simulink model "bh_proto_TQ_FFWD"  (R2016b)
settings: Solver=ode23s  StartTime=0.0  StopTime=60  FixedStep=0.001  RelTol=1e-5  EnableMultiTasking=on
undefined symbols (not defined in the file or in its folder): b1_damp, b2_damp, b3_damp, b4_damp, g, L1x, L1y, L1z, L2x, L2y, L2z, L3x, L3y, L3z, mass1, mass2, mass3, mass4, Rturn, TH1, TH1_D, TH1_DD, TH2, TH2_D, TH2_DD, TH3, TH3_D, TH3_DD, TH4, TH4_D, TH4_DD, theta1_0, theta1_dot_0, theta2_0, theta2_dot_0, theta3_0, theta3_dot_0, theta4_0, theta4_dot_0
libraries: simulink_extras x34, simulink x11, discretizing x8
(part 1 of 3)
settings Model: SimulationMode=rapid-accelerator  Creator=bhorton  LastModifiedBy=bhorton
settings SolverCC: ZeroCrossAlgorithm=Adaptive
settings OptimizationCC: LifeSpan=inf
settings DebuggingCC: SFUnexpectedBacktrackingDiag=warning  SFNoUnconditionalDefaultTransitionDiag=warning  SFExecutionAtInitializationDiag=none
settings GRTTargetCC: TargetLangStandard=C89/C90 (ANSI)
settings ConfigComp: CovMetricSettings=dw  CovHtmlReporting=on  CovSaveCumulativeToWorkspaceVar=on  CovSaveSingleToWorkspaceVar=on  CovExternalEMLEnable=off
settings SimscapeCC: SimscapeLogDataHistory=10000  SelectedTab=General

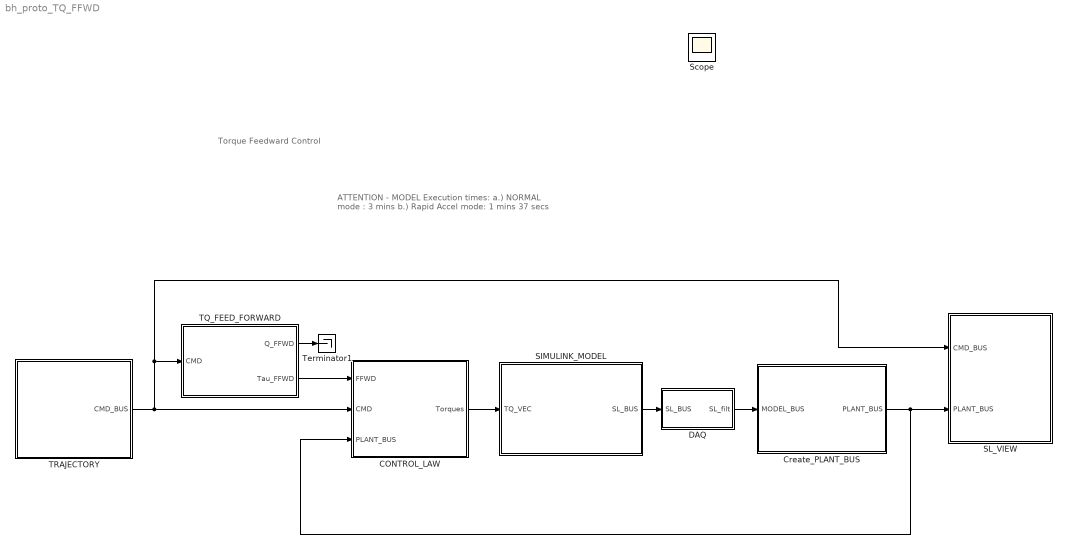
== system bh_proto_TQ_FFWD ==
  note: Torque Feedward Control
  note: ATTENTION - MODEL Execution times:
      | a.) NORMAL mode : 3 mins
      | b.) Rapid Accel mode: 1 mins 37 secs
  CONTROL_LAW : Subsystem
  Create_PLANT_BUS : Subsystem
  DAQ : Subsystem
  SIMULINK_MODEL : Subsystem
  SL_VIEW : Subsystem
  TQ_FEED_FORWARD : Subsystem
  TRAJECTORY : Subsystem
  Terminator1 : Terminator
  Scope : Scope
  wires:
  TRAJECTORY/1(CMD_BUS) -> SL_VIEW/1(CMD_BUS), TQ_FEED_FORWARD/1(CMD), CONTROL_LAW/2(CMD)
  Create_PLANT_BUS/1(PLANT_BUS) -> SL_VIEW/2(PLANT_BUS), CONTROL_LAW/3(PLANT_BUS)
  SIMULINK_MODEL/1(SL_BUS) -> DAQ/1(SL_BUS)
  CONTROL_LAW/1(Torques) -> SIMULINK_MODEL/1(TQ_VEC)
  TQ_FEED_FORWARD/2(Tau_FFWD) -> CONTROL_LAW/1(FFWD)
  TQ_FEED_FORWARD/1(Q_FFWD) -> Terminator1/1
  DAQ/1(SL_filt) -> Create_PLANT_BUS/1(MODEL_BUS)

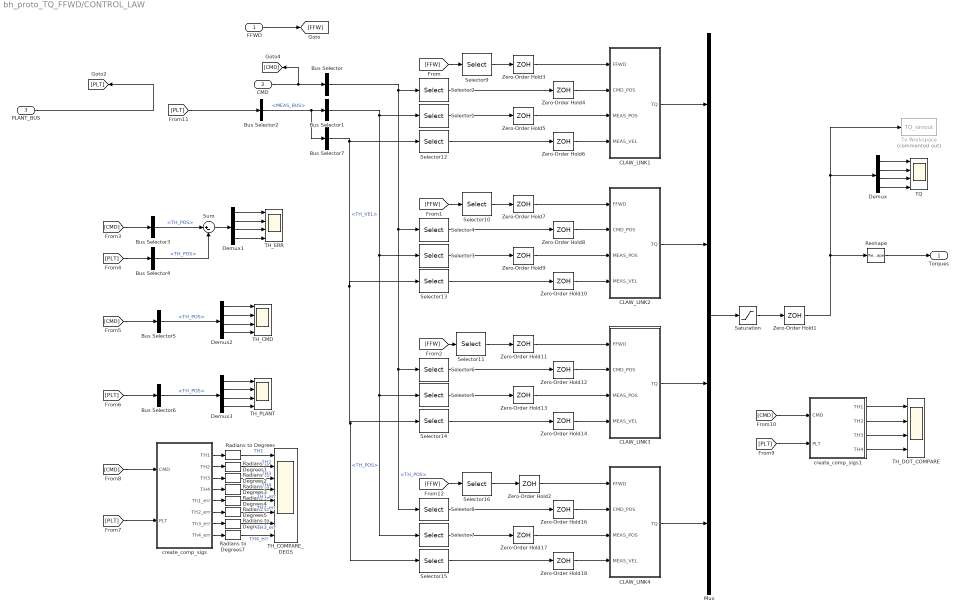
== system bh_proto_TQ_FFWD/CONTROL_LAW ==
  FFWD : Inport
  CMD : Inport  Port=2
  PLANT_BUS : Inport  Port=3
  Bus Selector{,1,3,5} (4 alike) : BusSelector  OutputSignals=TH_POS
  Bus Selector2 : BusSelector  OutputSignals=MEAS_BUS
  Bus Selector4 : BusSelector  OutputSignals=MEAS_BUS.TH_POS
  Bus Selector6 : BusSelector  OutputSignals=MEAS_BUS.TH_POS
  Bus Selector7 : BusSelector  OutputSignals=TH_VEL
  CLAW_LINK1 : Subsystem
  CLAW_LINK2 : Subsystem
  CLAW_LINK3 : Subsystem
  CLAW_LINK4 : Subsystem
  Demux{,1..3} (4 alike) : Demux
  Mux : Mux
  Radians to Degrees{,1..7} (8 alike) : simulink_extras/Transformations/Radians to Degrees
  Reshape : Reshape  OutputDimensionality=Column vector (2-D)
  Saturation : Saturate  UpperLimit=3  LowerLimit=-3
  Selector{1..2,9,12} (4 alike) : Selector  InputPortWidth=4  IndexOptions=Index vector (dialog)  Indices=1  OutputSizes=1
  Selector{3..4,10,13} (4 alike) : Selector  InputPortWidth=4  IndexOptions=Index vector (dialog)  Indices=2  OutputSizes=1
  Selector{5..6,11,14} (4 alike) : Selector  InputPortWidth=4  IndexOptions=Index vector (dialog)  Indices=3  OutputSizes=1
  Selector{7..8,15..16} (4 alike) : Selector  InputPortWidth=4  IndexOptions=Index vector (dialog)  Indices=4  OutputSizes=1
  Sum : Sum  Inputs=|+-
  TH_CMD : Scope  NumInputPorts=4
  TH_COMPARE_DEGS : Scope  NumInputPorts=8
  TH_DOT_COMPARE : Scope  NumInputPorts=4
  TH_ERR : Scope  NumInputPorts=4
  TH_PLANT : Scope  NumInputPorts=4
  TQ : Scope  NumInputPorts=4
  To Workspace : ToWorkspace  Commented=on  VariableName=TQ_simout  SaveFormat=Structure With Time  SampleTime=-1
  Zero-Order Hold{1..14,16..18} (17 alike) : ZeroOrderHold  SampleTime=0.001
      settings: AttributesFormatString=DT =%<SampleTime>
  create_comp_sigs : Subsystem
  create_comp_sigs1 : Subsystem
  Torques : Outport
  wires:
  Mux/1 -> Saturation/1
  Selector9/1 -> Zero-Order Hold3/1
  CMD/1 -> [CMD], Bus Selector/1
  Selector1/1 -> Zero-Order Hold5/1
  Selector2/1 -> Zero-Order Hold4/1
  Bus Selector/1 -> Selector8/1, Selector6/1, Selector4/1, Selector2/1  "<TH_POS>"
  Bus Selector1/1 -> Selector5/1, Selector7/1, Selector3/1, Selector1/1  "<TH_POS>"
  Bus Selector2/1 -> Bus Selector7/1, Bus Selector1/1  "<MEAS_BUS>"
  Demux/1 -> TQ/1
  Demux/2 -> TQ/2
  Demux/4 -> TQ/4
  Demux/3 -> TQ/3
  FFWD/1 -> [FFW]
  [FFW] -> Selector9/1
  [FFW] -> Selector10/1
  [FFW] -> Selector11/1
  Demux1/1 -> TH_ERR/1
  Demux1/2 -> TH_ERR/2
  Demux1/4 -> TH_ERR/4
  Demux1/3 -> TH_ERR/3
  PLANT_BUS/1 -> [PLT]
  [CMD] -> Bus Selector3/1
  [PLT] -> Bus Selector4/1
  Bus Selector3/1 -> Sum/1  "<TH_POS>"
  Bus Selector4/1 -> Sum/2  "<TH_POS>"
  Sum/1 -> Demux1/1
  Demux2/1 -> TH_CMD/1
  Demux2/2 -> TH_CMD/2
  Demux2/4 -> TH_CMD/4
  Demux2/3 -> TH_CMD/3
  [CMD] -> Bus Selector5/1
  Bus Selector5/1 -> Demux2/1  "<TH_POS>"
  Demux3/1 -> TH_PLANT/1
  Demux3/2 -> TH_PLANT/2
  Demux3/4 -> TH_PLANT/4
  Demux3/3 -> TH_PLANT/3
  [PLT] -> Bus Selector6/1
  Bus Selector6/1 -> Demux3/1  "<TH_POS>"
  Bus Selector7/1 -> Selector15/1, Selector14/1, Selector13/1, Selector12/1  "<TH_VEL>"
  Selector12/1 -> Zero-Order Hold6/1
  CLAW_LINK4/1(TQ) -> Mux/4
  CLAW_LINK3/1(TQ) -> Mux/3
  CLAW_LINK2/1(TQ) -> Mux/2
  CLAW_LINK1/1(TQ) -> Mux/1
  Saturation/1 -> Zero-Order Hold1/1
  Zero-Order Hold3/1 -> CLAW_LINK1/1(FFWD)
  Zero-Order Hold4/1 -> CLAW_LINK1/2(CMD_POS)
  Zero-Order Hold5/1 -> CLAW_LINK1/3(MEAS_POS)
  Zero-Order Hold6/1 -> CLAW_LINK1/4(MEAS_VEL)
  Selector10/1 -> Zero-Order Hold7/1
  Selector3/1 -> Zero-Order Hold9/1
  Selector4/1 -> Zero-Order Hold8/1
  Selector13/1 -> Zero-Order Hold10/1
  Zero-Order Hold7/1 -> CLAW_LINK2/1(FFWD)
  Zero-Order Hold8/1 -> CLAW_LINK2/2(CMD_POS)
  Zero-Order Hold9/1 -> CLAW_LINK2/3(MEAS_POS)
  Zero-Order Hold10/1 -> CLAW_LINK2/4(MEAS_VEL)
  Selector5/1 -> Zero-Order Hold13/1
  Selector6/1 -> Zero-Order Hold12/1
  Selector14/1 -> Zero-Order Hold14/1
  Zero-Order Hold11/1 -> CLAW_LINK3/1(FFWD)
  Zero-Order Hold12/1 -> CLAW_LINK3/2(CMD_POS)
  Zero-Order Hold13/1 -> CLAW_LINK3/3(MEAS_POS)
  Zero-Order Hold14/1 -> CLAW_LINK3/4(MEAS_VEL)
  Selector11/1 -> Zero-Order Hold11/1
  Selector7/1 -> Zero-Order Hold17/1
  Selector8/1 -> Zero-Order Hold16/1
  Selector15/1 -> Zero-Order Hold18/1
  Zero-Order Hold16/1 -> CLAW_LINK4/2(CMD_POS)
  Zero-Order Hold17/1 -> CLAW_LINK4/3(MEAS_POS)
  Zero-Order Hold18/1 -> CLAW_LINK4/4(MEAS_VEL)
  Zero-Order Hold2/1 -> CLAW_LINK4/1(FFWD)
  [PLT] -> create_comp_sigs/2(PLT)
  [CMD] -> create_comp_sigs/1(CMD)
  create_comp_sigs/1(TH1) -> Radians to Degrees/1
  create_comp_sigs/2(TH2) -> Radians to Degrees1/1
  create_comp_sigs/3(TH3) -> Radians to Degrees2/1
  create_comp_sigs/4(TH4) -> Radians to Degrees3/1
  [PLT] -> create_comp_sigs1/2(PLT)
  [CMD] -> create_comp_sigs1/1(CMD)
  create_comp_sigs1/1(TH1) -> TH_DOT_COMPARE/1
  create_comp_sigs1/2(TH2) -> TH_DOT_COMPARE/2
  create_comp_sigs1/3(TH3) -> TH_DOT_COMPARE/3
  create_comp_sigs1/4(TH4) -> TH_DOT_COMPARE/4
  Zero-Order Hold1/1 -> Reshape/1, To Workspace/1, Demux/1
  [PLT] -> Bus Selector2/1
  [FFW] -> Selector16/1
  Selector16/1 -> Zero-Order Hold2/1
  create_comp_sigs/5(Th1_err) -> Radians to Degrees4/1
  create_comp_sigs/6(TH2_err) -> Radians to Degrees5/1
  create_comp_sigs/7(Th3_err) -> Radians to Degrees6/1
  create_comp_sigs/8(Th4_err) -> Radians to Degrees7/1
  Radians to Degrees7/1 -> TH_COMPARE_DEGS/8  "TH4_err"
  Radians to Degrees6/1 -> TH_COMPARE_DEGS/7  "TH3_err"
  Radians to Degrees5/1 -> TH_COMPARE_DEGS/6  "TH2_err"
  Radians to Degrees4/1 -> TH_COMPARE_DEGS/5  "TH1_err"
  Radians to Degrees3/1 -> TH_COMPARE_DEGS/4  "TH4"
  Radians to Degrees2/1 -> TH_COMPARE_DEGS/3  "TH3"
  Radians to Degrees1/1 -> TH_COMPARE_DEGS/2  "TH2"
  Radians to Degrees/1 -> TH_COMPARE_DEGS/1  "TH1"
  Reshape/1 -> Torques/1

== system bh_proto_TQ_FFWD/Create_PLANT_BUS ==
  MODEL_BUS : Inport
  CALC_BUS : Subsystem
  MEAS : Subsystem
  Subsystem : Subsystem
  Subsystem1 : Subsystem
  PLANT_BUS : Outport
  wires:
  MODEL_BUS/1 -> MEAS/1(MODEL_BUS), CALC_BUS/1(MODEL_BUS), Subsystem/1(MODEL)
  Subsystem/1(PLANT_B) -> PLANT_BUS/1
  CALC_BUS/1(CALC_POS) -> Subsystem1/1(POS), Subsystem/3(CALC_POS)
  MEAS/1(MEAS) -> Subsystem/2(MEAS)
  Subsystem1/1(GTQ) -> Subsystem/4(CALC_GRAV_TQ)

== system bh_proto_TQ_FFWD/DAQ ==
  SL_BUS : Inport
  Bus Assignment : BusAssignment  AssignedSignals=TH1,TH2,TH3,TH4,TH1_D,TH2_D,TH3_D,TH4_D,TH1_DD,TH2_DD,TH3_DD,TH4_DD
  Bus Selector : BusSelector  OutputSignals=TH1,TH2,TH3,TH4
  Bus Selector1 : BusSelector  OutputSignals=TH1_D,TH2_D,TH3_D,TH4_D
  Bus Selector2 : BusSelector  OutputSignals=TH1_DD,TH2_DD,TH3_DD,TH4_DD
  Demux : Demux
  Demux1 : Demux
  Demux2 : Demux
  LPF : Subsystem  mask{fc=100}
      mask prompts: fc "LPF cutoff Frequency (Hz)"
      mask Display: fprintf('LPF\n fc = %.0f (Hz)', fc);
  Mux : Mux
  Mux1 : Mux
  Mux2 : Mux
  SL_filt : Outport
  wires:
  Bus Selector/1 -> Mux/1  "<TH1>"
  Bus Selector/2 -> Mux/2  "<TH2>"
  Bus Selector/3 -> Mux/3  "<TH3>"
  Bus Selector/4 -> Mux/4  "<TH4>"
  Bus Selector1/1 -> Mux1/1  "<TH1_D>"
  Bus Selector1/2 -> Mux1/2  "<TH2_D>"
  Bus Selector1/3 -> Mux1/3  "<TH3_D>"
  Bus Selector1/4 -> Mux1/4  "<TH4_D>"
  Bus Selector2/1 -> Mux2/1  "<TH1_DD>"
  Bus Selector2/2 -> Mux2/2  "<TH2_DD>"
  Bus Selector2/3 -> Mux2/3  "<TH3_DD>"
  Bus Selector2/4 -> Mux2/4  "<TH4_DD>"
  Mux1/1 -> LPF/2(TH_D)
  Mux/1 -> LPF/1(TH)
  Mux2/1 -> LPF/3(TH_DD)
  LPF/1(TH_filt) -> Demux/1
  LPF/2(TH_D_filt) -> Demux1/1
  LPF/3(TH_DD_filt) -> Demux2/1
  SL_BUS/1 -> [A], Bus Selector2/1, Bus Selector/1, Bus Selector1/1
  [A] -> Bus Assignment/1
  Demux/1 -> Bus Assignment/2
  Demux/2 -> Bus Assignment/3
  Demux/3 -> Bus Assignment/4
  Demux/4 -> Bus Assignment/5
  Demux1/1 -> Bus Assignment/6
  Demux1/2 -> Bus Assignment/7
  Demux1/3 -> Bus Assignment/8
  Demux1/4 -> Bus Assignment/9
  Demux2/1 -> Bus Assignment/10
  Demux2/2 -> Bus Assignment/11
  Demux2/3 -> Bus Assignment/12
  Demux2/4 -> Bus Assignment/13
  Bus Assignment/1 -> SL_filt/1

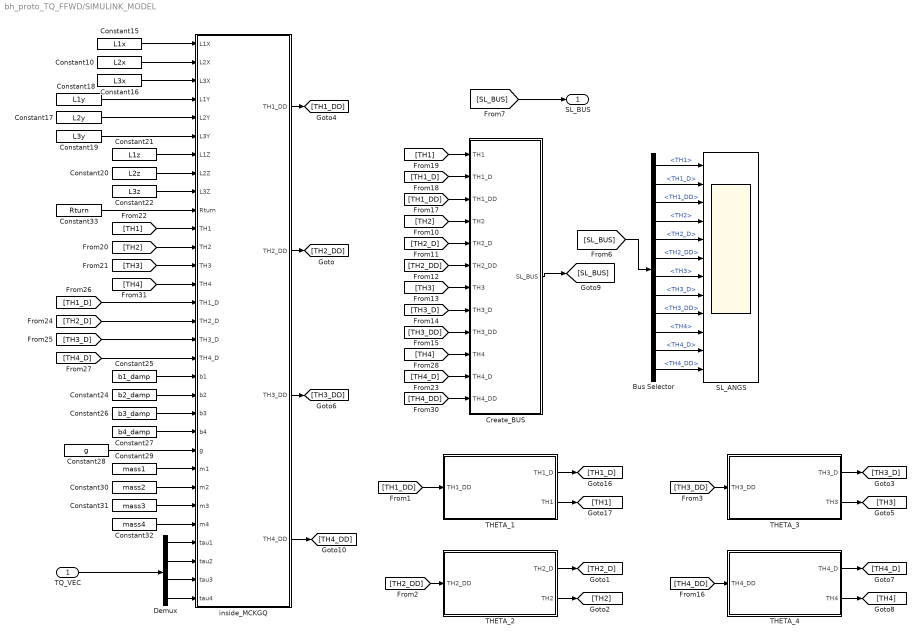
== system bh_proto_TQ_FFWD/SIMULINK_MODEL ==
  TQ_VEC : Inport
  Bus Selector : BusSelector  OutputSignals=TH1,TH1_D,TH1_DD,TH2,TH2_D,TH2_DD,TH3,TH3_D,TH3_DD,TH4,TH4_D,TH4_DD
  Constant10 : Constant  Value=L2x
  Constant15 : Constant  Value=L1x
  Constant16 : Constant  Value=L3x
  Constant17 : Constant  Value=L2y
  Constant18 : Constant  Value=L1y
  Constant19 : Constant  Value=L3y
  Constant20 : Constant  Value=L2z
  Constant21 : Constant  Value=L1z
  Constant22 : Constant  Value=L3z
  Constant24 : Constant  Value=b2_damp
  Constant25 : Constant  Value=b1_damp
  Constant26 : Constant  Value=b3_damp
  Constant27 : Constant  Value=b4_damp
  Constant28 : Constant  Value=g
  Constant29 : Constant  Value=mass1
  Constant30 : Constant  Value=mass2
  Constant31 : Constant  Value=mass3
  Constant32 : Constant  Value=mass4
  Constant33 : Constant  Value=Rturn
  Create_BUS : Subsystem
  Demux : Demux
  SL_ANGS : Scope  NumInputPorts=12
  THETA_1 : Subsystem
  THETA_2 : Subsystem
  THETA_3 : Subsystem
  THETA_4 : Subsystem
  inside_MCKGQ : Subsystem
  SL_BUS : Outport
  wires:
  [SL_BUS] -> Bus Selector/1
  [SL_BUS] -> SL_BUS/1
  Create_BUS/1(SL_BUS) -> [SL_BUS]
  Bus Selector/2 -> SL_ANGS/2  "<TH1_D>"
  Bus Selector/3 -> SL_ANGS/3  "<TH1_DD>"
  Bus Selector/1 -> SL_ANGS/1  "<TH1>"
  Bus Selector/4 -> SL_ANGS/4  "<TH2>"
  Bus Selector/5 -> SL_ANGS/5  "<TH2_D>"
  Bus Selector/6 -> SL_ANGS/6  "<TH2_DD>"
  Bus Selector/7 -> SL_ANGS/7  "<TH3>"
  Bus Selector/8 -> SL_ANGS/8  "<TH3_D>"
  Bus Selector/9 -> SL_ANGS/9  "<TH3_DD>"
  [TH2_DD] -> THETA_2/1(TH2_DD)
  THETA_2/2(TH2) -> [TH2]
  THETA_2/1(TH2_D) -> [TH2_D]
  [TH1_DD] -> THETA_1/1(TH1_DD)
  THETA_1/1(TH1_D) -> [TH1_D]
  THETA_1/2(TH1) -> [TH1]
  inside_MCKGQ/2(TH2_DD) -> [TH2_DD]
  [TH3_DD] -> THETA_3/1(TH3_DD)
  THETA_3/2(TH3) -> [TH3]
  THETA_3/1(TH3_D) -> [TH3_D]
  inside_MCKGQ/1(TH1_DD) -> [TH1_DD]
  inside_MCKGQ/3(TH3_DD) -> [TH3_DD]
  [TH3_DD] -> Create_BUS/9(TH3_DD)
  [TH1] -> Create_BUS/1(TH1)
  [TH1_D] -> Create_BUS/2(TH1_D)
  [TH1_DD] -> Create_BUS/3(TH1_DD)
  [TH2] -> Create_BUS/4(TH2)
  [TH2_D] -> Create_BUS/5(TH2_D)
  [TH2_DD] -> Create_BUS/6(TH2_DD)
  [TH3] -> Create_BUS/7(TH3)
  [TH3_D] -> Create_BUS/8(TH3_D)
  [TH4_DD] -> THETA_4/1(TH4_DD)
  THETA_4/2(TH4) -> [TH4]
  THETA_4/1(TH4_D) -> [TH4_D]
  [TH2] -> inside_MCKGQ/12(TH2)
  [TH3] -> inside_MCKGQ/13(TH3)
  [TH1] -> inside_MCKGQ/11(TH1)
  Constant10/1 -> inside_MCKGQ/2(L2X)
  Constant16/1 -> inside_MCKGQ/3(L3X)
  Constant15/1 -> inside_MCKGQ/1(L1X)
  Constant19/1 -> inside_MCKGQ/6(L3Y)
  Constant17/1 -> inside_MCKGQ/5(L2Y)
  Constant18/1 -> inside_MCKGQ/4(L1Y)
  Constant22/1 -> inside_MCKGQ/9(L3Z)
  Constant20/1 -> inside_MCKGQ/8(L2Z)
  Constant21/1 -> inside_MCKGQ/7(L1Z)
  [TH1_D] -> inside_MCKGQ/15(TH1_D)
  [TH2_D] -> inside_MCKGQ/16(TH2_D)
  [TH3_D] -> inside_MCKGQ/17(TH3_D)
  [TH4_D] -> inside_MCKGQ/18(TH4_D)
  Constant25/1 -> inside_MCKGQ/19(b1)
  Constant24/1 -> inside_MCKGQ/20(b2)
  Constant26/1 -> inside_MCKGQ/21(b3)
  Constant27/1 -> inside_MCKGQ/22(b4)
  Constant28/1 -> inside_MCKGQ/23(g)
  Constant29/1 -> inside_MCKGQ/24(m1)
  Constant30/1 -> inside_MCKGQ/25(m2)
  Constant31/1 -> inside_MCKGQ/26(m3)
  Constant32/1 -> inside_MCKGQ/27(m4)
  Constant33/1 -> inside_MCKGQ/10(Rturn)
  [TH4_D] -> Create_BUS/11(TH4_D)
  [TH4_DD] -> Create_BUS/12(TH4_DD)
  [TH4] -> Create_BUS/10(TH4)
  [TH4] -> inside_MCKGQ/14(TH4)
  inside_MCKGQ/4(TH4_DD) -> [TH4_DD]
  Bus Selector/10 -> SL_ANGS/10  "<TH4>"
  Bus Selector/11 -> SL_ANGS/11  "<TH4_D>"
  Bus Selector/12 -> SL_ANGS/12  "<TH4_DD>"
  Demux/2 -> inside_MCKGQ/29(tau2)
  Demux/3 -> inside_MCKGQ/30(tau3)
  Demux/4 -> inside_MCKGQ/31(tau4)
  TQ_VEC/1 -> Demux/1
  Demux/1 -> inside_MCKGQ/28(tau1)

== system bh_proto_TQ_FFWD/SL_VIEW ==
  CMD_BUS : Inport
  PLANT_BUS : Inport  Port=2
  Bus Selector4 : BusSelector  OutputSignals=CALC_POS_BUS.WF_pos_EFF
  COMPARE_XYZ_EFF (mm) COMPARE_THETA (degs) : Scope  NumInputPorts=16
  Demux : Demux  Outputs=3
  Gain{,1..5} (6 alike) : Gain  Gain=1000
  Ground : Ground
  Ground1 : Ground
  MODEL_MATH_SL : simulink/Sinks/XY Graph  xmin=0  xmax=1.6  ymin=0  ymax=1.6  st=-1
  PLANT_XYZ_EFF : Scope  NumInputPorts=3
  Radians to Degrees{,1..7} (8 alike) : simulink_extras/Transformations/Radians to Degrees
  XYZ_EFF_COMPARE : Subsystem
  create_comp_sigs : Subsystem
  wires:
  CMD_BUS/1 -> [CMD]
  PLANT_BUS/1 -> [PLT]
  [CMD] -> XYZ_EFF_COMPARE/1(CMD_BUS)
  [PLT] -> XYZ_EFF_COMPARE/2(PLANT_BUS)
  XYZ_EFF_COMPARE/1(X) -> Gain/1
  XYZ_EFF_COMPARE/2(Y) -> Gain2/1
  XYZ_EFF_COMPARE/3(Z) -> Gain1/1
  Bus Selector4/1 -> Demux/1  "<WF_pos_EFF>"
  Demux/1 -> MODEL_MATH_SL/1, PLANT_XYZ_EFF/1
  Demux/2 -> MODEL_MATH_SL/2, PLANT_XYZ_EFF/2
  [PLT] -> Bus Selector4/1
  Demux/3 -> PLANT_XYZ_EFF/3
  Gain/1 -> COMPARE_XYZ_EFF (mm) COMPARE_THETA (degs)/1  "X_mm"
  Gain1/1 -> COMPARE_XYZ_EFF (mm) COMPARE_THETA (degs)/3  "Z_mm"
  Gain2/1 -> COMPARE_XYZ_EFF (mm) COMPARE_THETA (degs)/2  "Y_mm"
  Gain3/1 -> COMPARE_XYZ_EFF (mm) COMPARE_THETA (degs)/5  "Xerr_mm"
  Gain4/1 -> COMPARE_XYZ_EFF (mm) COMPARE_THETA (degs)/6  "Yerr_mm"
  Gain5/1 -> COMPARE_XYZ_EFF (mm) COMPARE_THETA (degs)/7  "Zerr_mm"
  XYZ_EFF_COMPARE/6(Zerr) -> Gain5/1
  XYZ_EFF_COMPARE/5(Yerr) -> Gain4/1
  XYZ_EFF_COMPARE/4(Xerr) -> Gain3/1
  [PLT] -> create_comp_sigs/2(PLT)
  [CMD] -> create_comp_sigs/1(CMD)
  create_comp_sigs/1(TH1) -> Radians to Degrees/1
  create_comp_sigs/2(TH2) -> Radians to Degrees1/1
  create_comp_sigs/3(TH3) -> Radians to Degrees2/1
  create_comp_sigs/4(TH4) -> Radians to Degrees3/1
  create_comp_sigs/5(Th1_err) -> Radians to Degrees4/1
  create_comp_sigs/6(TH2_err) -> Radians to Degrees5/1
  create_comp_sigs/7(Th3_err) -> Radians to Degrees6/1
  create_comp_sigs/8(Th4_err) -> Radians to Degrees7/1
  Radians to Degrees7/1 -> COMPARE_XYZ_EFF (mm) COMPARE_THETA (degs)/16  "TH4_err_deg"
  Radians to Degrees6/1 -> COMPARE_XYZ_EFF (mm) COMPARE_THETA (degs)/15  "TH3_err_deg"
  Radians to Degrees5/1 -> COMPARE_XYZ_EFF (mm) COMPARE_THETA (degs)/14  "TH2_err_deg"
  Radians to Degrees4/1 -> COMPARE_XYZ_EFF (mm) COMPARE_THETA (degs)/13  "TH1_err_deg"
  Radians to Degrees3/1 -> COMPARE_XYZ_EFF (mm) COMPARE_THETA (degs)/12  "TH4_deg"
  Radians to Degrees2/1 -> COMPARE_XYZ_EFF (mm) COMPARE_THETA (degs)/11  "TH3_deg"
  Radians to Degrees1/1 -> COMPARE_XYZ_EFF (mm) COMPARE_THETA (degs)/10  "TH2_deg"
  Radians to Degrees/1 -> COMPARE_XYZ_EFF (mm) COMPARE_THETA (degs)/9  "TH1_deg"
  Ground/1 -> COMPARE_XYZ_EFF (mm) COMPARE_THETA (degs)/4
  Ground1/1 -> COMPARE_XYZ_EFF (mm) COMPARE_THETA (degs)/8

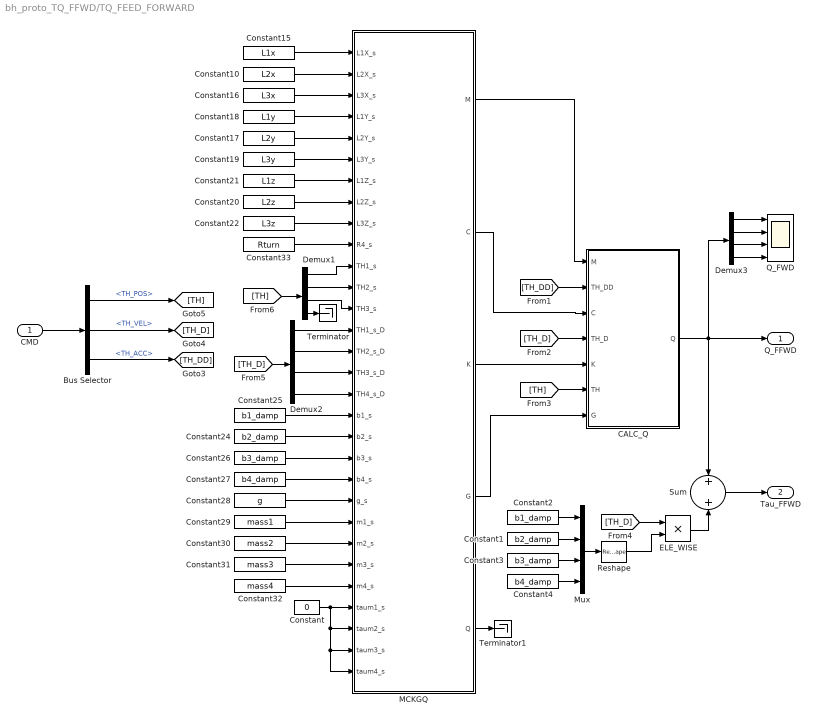
== system bh_proto_TQ_FFWD/TQ_FEED_FORWARD ==
  CMD : Inport
  Bus Selector : BusSelector  OutputSignals=TH_POS,TH_VEL,TH_ACC
  CALC_Q : Subsystem
  Constant : Constant  Value=0
  Constant1 : Constant  Value=b2_damp
  Constant10 : Constant  Value=L2x
  Constant15 : Constant  Value=L1x
  Constant16 : Constant  Value=L3x
  Constant17 : Constant  Value=L2y
  Constant18 : Constant  Value=L1y
  Constant19 : Constant  Value=L3y
  Constant2 : Constant  Value=b1_damp
  Constant20 : Constant  Value=L2z
  Constant21 : Constant  Value=L1z
  Constant22 : Constant  Value=L3z
  Constant24 : Constant  Value=b2_damp
  Constant25 : Constant  Value=b1_damp
  Constant26 : Constant  Value=b3_damp
  Constant27 : Constant  Value=b4_damp
  Constant28 : Constant  Value=g
  Constant29 : Constant  Value=mass1
  Constant3 : Constant  Value=b3_damp
  Constant30 : Constant  Value=mass2
  Constant31 : Constant  Value=mass3
  Constant32 : Constant  Value=mass4
  Constant33 : Constant  Value=Rturn
  Constant4 : Constant  Value=b4_damp
  Demux1 : Demux
  Demux2 : Demux
  Demux3 : Demux
  ELE_WISE : Product
  MCKGQ : MATLAB Function  TreatAsAtomicUnit=on
  Mux : Mux
  Q_FWD : Scope  NumInputPorts=4
  Reshape : Reshape  OutputDimensionality=Column vector (2-D)
  Sum : Sum  Inputs=+|+
  Terminator : Terminator
  Terminator1 : Terminator
  Q_FFWD : Outport
  Tau_FFWD : Outport  Port=2
  wires:
  Bus Selector/1 -> [TH]  "<TH_POS>"
  Bus Selector/3 -> [TH_DD]  "<TH_ACC>"
  CMD/1 -> Bus Selector/1
  Bus Selector/2 -> [TH_D]  "<TH_VEL>"
  Constant10/1 -> MCKGQ/2(L2X_s)
  Constant16/1 -> MCKGQ/3(L3X_s)
  Constant15/1 -> MCKGQ/1(L1X_s)
  Constant19/1 -> MCKGQ/6(L3Y_s)
  Constant17/1 -> MCKGQ/5(L2Y_s)
  Constant18/1 -> MCKGQ/4(L1Y_s)
  Constant22/1 -> MCKGQ/9(L3Z_s)
  Constant20/1 -> MCKGQ/8(L2Z_s)
  Constant21/1 -> MCKGQ/7(L1Z_s)
  Constant25/1 -> MCKGQ/18(b1_s)
  Constant24/1 -> MCKGQ/19(b2_s)
  Constant26/1 -> MCKGQ/20(b3_s)
  Constant27/1 -> MCKGQ/21(b4_s)
  Constant28/1 -> MCKGQ/22(g_s)
  Constant29/1 -> MCKGQ/23(m1_s)
  Constant30/1 -> MCKGQ/24(m2_s)
  Constant31/1 -> MCKGQ/25(m3_s)
  Constant32/1 -> MCKGQ/26(m4_s)
  Constant33/1 -> MCKGQ/10(R4_s)
  Constant/1 -> MCKGQ/28(taum2_s), MCKGQ/29(taum3_s), MCKGQ/30(taum4_s), MCKGQ/27(taum1_s)
  Demux1/2 -> MCKGQ/12(TH2_s)
  Demux1/1 -> MCKGQ/11(TH1_s)
  Demux1/3 -> MCKGQ/13(TH3_s)
  Demux1/4 -> Terminator/1
  Demux2/1 -> MCKGQ/14(TH1_s_D)
  Demux2/2 -> MCKGQ/15(TH2_s_D)
  Demux2/3 -> MCKGQ/16(TH3_s_D)
  Demux2/4 -> MCKGQ/17(TH4_s_D)
  MCKGQ/3(K) -> CALC_Q/5(K)
  MCKGQ/2(C) -> CALC_Q/3(C)
  MCKGQ/1(M) -> CALC_Q/1(M)
  MCKGQ/4(G) -> CALC_Q/7(G)
  MCKGQ/5(Q) -> Terminator1/1
  [TH] -> CALC_Q/6(TH)
  [TH_D] -> CALC_Q/4(TH_D)
  CALC_Q/1(Q) -> Demux3/1, Sum/1, Q_FFWD/1
  Demux3/1 -> Q_FWD/1
  Demux3/3 -> Q_FWD/3
  Demux3/4 -> Q_FWD/4
  Demux3/2 -> Q_FWD/2
  [TH_DD] -> CALC_Q/2(TH_DD)
  Constant2/1 -> Mux/1
  Constant1/1 -> Mux/2
  Constant3/1 -> Mux/3
  Constant4/1 -> Mux/4
  Mux/1 -> Reshape/1
  [TH_D] -> ELE_WISE/1
  Reshape/1 -> ELE_WISE/2
  ELE_WISE/1 -> Sum/2
  Sum/1 -> Tau_FFWD/1
  [TH] -> Demux1/1
  [TH_D] -> Demux2/1

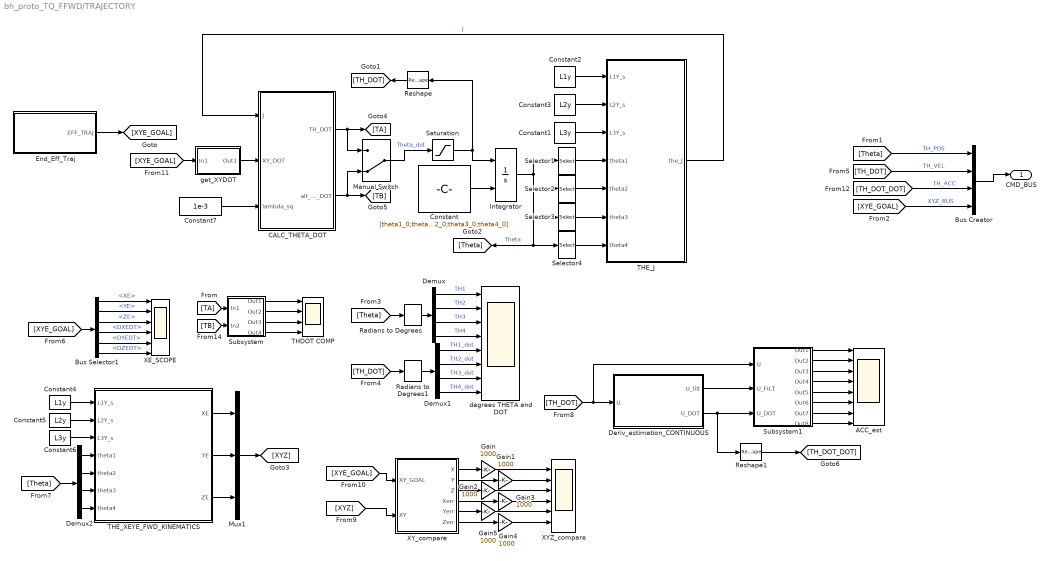
== system bh_proto_TQ_FFWD/TRAJECTORY ==
  ACC_est : Scope  NumInputPorts=8
  Bus Creator : BusCreator  Inputs=4
  Bus Selector1 : BusSelector  OutputSignals=XE,YE,ZE,DXEDT,DYEDT,DZEDT
  CALC_THETA_DOT : MATLAB Function  TreatAsAtomicUnit=on
  Constant : Constant  Value=[theta1_0;theta2_0;theta3_0;theta4_0]  VectorParams1D=off
  Constant1 : Constant  Value=L3y
  Constant2 : Constant  Value=L1y
  Constant3 : Constant  Value=L2y
  Constant4 : Constant  Value=L1y
  Constant5 : Constant  Value=L2y
  Constant6 : Constant  Value=L3y
  Constant7 : Constant  Value=1e-3
  Demux : Demux
  Demux1 : Demux
  Demux2 : Demux
  Deriv_estimation_CONTINUOUS : Subsystem  mask(Derivative Estimation){wn=2*pi*100, p=1, x0_val=0, v0_val=0}
      mask prompts: wn "Natural frequency, wn (rad/sec)"; p "Damping ratio, p"; x0_val "X_IC"; v0_val "X_DOT_IC"
      mask help:
      | A simple derivative estimator using a 2nd order representation between input and output.
      |
      | The integrators use a discrete FORWARd Euler rule, and a sample time needs to be specified.
      mask init:
      | str0 = sprintf('fn = %.2f [Hz]', (wn/(2*pi)));
      | str1 = sprintf('wn = %.2f', wn);
      | str2 = sprintf('p  = %.3g', p);
      | %str3 = sprintf('dt = %.2g', dt);
      | str = char(str0,str1,str2);
      mask Display: disp(str)
  End_Eff_Traj : Subsystem
  Gain{,1..5} (6 alike) : Gain  Gain=1000
  Integrator : Integrator  InitialConditionSource=external
  Manual Switch : ManualSwitch  CurrentSetting=0
  Mux1 : Mux  Inputs=3
  Radians to Degrees : simulink_extras/Transformations/Radians to Degrees
  Radians to Degrees1 : simulink_extras/Transformations/Radians to Degrees
  Reshape : Reshape  OutputDimensionality=Column vector (2-D)
  Reshape1 : Reshape  OutputDimensionality=Column vector (2-D)
  Saturation : Saturate  UpperLimit=6  LowerLimit=-6
  Selector1 : Selector  InputPortWidth=4  IndexOptions=Index vector (dialog)  Indices=1  OutputSizes=1
  Selector2 : Selector  InputPortWidth=4  IndexOptions=Index vector (dialog)  Indices=2  OutputSizes=1
  Selector3 : Selector  InputPortWidth=4  IndexOptions=Index vector (dialog)  Indices=3  OutputSizes=1
  Selector4 : Selector  InputPortWidth=4  IndexOptions=Index vector (dialog)  Indices=4  OutputSizes=1
  Subsystem : Subsystem
  Subsystem1 : Subsystem
  THDOT COMP : Scope  NumInputPorts=4
  THE_J : MATLAB Function  TreatAsAtomicUnit=on
  THE_XEYE_FWD_KINEMATICS : MATLAB Function  TreatAsAtomicUnit=on
  XE_SCOPE : Scope  NumInputPorts=6
  XYZ_compare : Scope  NumInputPorts=6
  XY_compare : Subsystem
  degrees THETA and DOT : Scope  NumInputPorts=8
  get_XYDOT : Subsystem
  CMD_BUS : Outport
  wires:
  Bus Selector1/1 -> XE_SCOPE/1  "<XE>"
  Bus Selector1/2 -> XE_SCOPE/2  "<YE>"
  Bus Selector1/3 -> XE_SCOPE/3  "<ZE>"
  Bus Selector1/4 -> XE_SCOPE/4  "<DXEDT>"
  Bus Selector1/5 -> XE_SCOPE/5  "<DYEDT>"
  Bus Selector1/6 -> XE_SCOPE/6  "<DZEDT>"
  [XYE_GOAL] -> Bus Selector1/1
  Constant/1 -> Integrator/2
  THE_J/1(the_J) -> CALC_THETA_DOT/1(J)  "J"
  get_XYDOT/1(Out1) -> CALC_THETA_DOT/2(XY_DOT)
  Manual Switch/1 -> Saturation/1  "Theta_dot"
  Integrator/1 -> Selector4/1, [Theta], Selector3/1, Selector2/1, Selector1/1  "Theta"
  [XYE_GOAL] -> get_XYDOT/1(In1)
  Saturation/1 -> Integrator/1, Reshape/1
  Selector4/1 -> THE_J/7(theta4)
  Selector3/1 -> THE_J/6(theta3)
  Selector2/1 -> THE_J/5(theta2)
  Selector1/1 -> THE_J/4(theta1)
  Constant2/1 -> THE_J/1(L1Y_s)
  Constant3/1 -> THE_J/2(L2Y_s)
  Constant1/1 -> THE_J/3(L3Y_s)
  CALC_THETA_DOT/1(TH_DOT) -> [TA], Manual Switch/1
  CALC_THETA_DOT/2(alt_TH_DOT) -> [TB], Manual Switch/2
  Constant7/1 -> CALC_THETA_DOT/3(lambda_sq)
  [TB] -> Subsystem/2(In2)
  [TA] -> Subsystem/1(In1)
  Subsystem/1(Out1) -> THDOT COMP/1
  Subsystem/2(Out2) -> THDOT COMP/2
  Subsystem/3(Out3) -> THDOT COMP/3
  Subsystem/4(Out4) -> THDOT COMP/4
  End_Eff_Traj/1(EFF_TRAJ) -> [XYE_GOAL]
  [TH_DOT] -> Bus Creator/2  "TH_VEL"
  [Theta] -> Bus Creator/1  "TH_POS"
  Bus Creator/1 -> CMD_BUS/1
  Reshape/1 -> [TH_DOT]
  [XYE_GOAL] -> Bus Creator/4  "XYZ_BUS"
  Demux/4 -> degrees THETA and DOT/4  "TH4"
  Demux/3 -> degrees THETA and DOT/3  "TH3"
  Demux/2 -> degrees THETA and DOT/2  "TH2"
  Demux/1 -> degrees THETA and DOT/1  "TH1"
  Demux1/1 -> degrees THETA and DOT/5  "TH1_dot"
  Demux1/2 -> degrees THETA and DOT/6  "TH2_dot"
  Demux1/3 -> degrees THETA and DOT/7  "TH3_dot"
  Demux1/4 -> degrees THETA and DOT/8  "TH4_dot"
  [Theta] -> Radians to Degrees/1
  Radians to Degrees/1 -> Demux/1
  [TH_DOT] -> Radians to Degrees1/1
  Radians to Degrees1/1 -> Demux1/1
  Constant4/1 -> THE_XEYE_FWD_KINEMATICS/1(L1Y_s)
  Constant6/1 -> THE_XEYE_FWD_KINEMATICS/3(L3Y_s)
  Constant5/1 -> THE_XEYE_FWD_KINEMATICS/2(L2Y_s)
  Demux2/1 -> THE_XEYE_FWD_KINEMATICS/4(theta1)
  Demux2/2 -> THE_XEYE_FWD_KINEMATICS/5(theta2)
  Demux2/3 -> THE_XEYE_FWD_KINEMATICS/6(theta3)
  Demux2/4 -> THE_XEYE_FWD_KINEMATICS/7(theta4)
  [Theta] -> Demux2/1
  THE_XEYE_FWD_KINEMATICS/1(XE) -> Mux1/1
  THE_XEYE_FWD_KINEMATICS/3(ZE) -> Mux1/3
  THE_XEYE_FWD_KINEMATICS/2(YE) -> Mux1/2
  Mux1/1 -> [XYZ]
  [XYZ] -> XY_compare/2(XY)
  [XYE_GOAL] -> XY_compare/1(XY_GOAL)
  [TH_DOT] -> Subsystem1/1(U), Deriv_estimation_CONTINUOUS/1(U)
  Subsystem1/1(Out1) -> ACC_est/1
  Subsystem1/2(Out2) -> ACC_est/2
  Subsystem1/3(Out3) -> ACC_est/3
  Subsystem1/4(Out4) -> ACC_est/4
  Subsystem1/5(Out5) -> ACC_est/5
  Subsystem1/6(Out6) -> ACC_est/6
  Subsystem1/7(Out7) -> ACC_est/7
  Subsystem1/8(Out8) -> ACC_est/8
  Deriv_estimation_CONTINUOUS/1(U_filt) -> Subsystem1/2(U_FILT)
  Deriv_estimation_CONTINUOUS/2(U_DOT) -> Reshape1/1, Subsystem1/3(U_DOT)
  [TH_DOT_DOT] -> Bus Creator/3  "TH_ACC"
  Reshape1/1 -> [TH_DOT_DOT]
  Gain/1 -> XYZ_compare/1
  Gain1/1 -> XYZ_compare/2
  Gain2/1 -> XYZ_compare/3
  XY_compare/1(X) -> Gain/1
  XY_compare/2(Y) -> Gain1/1
  XY_compare/3(Z) -> Gain2/1
  Gain4/1 -> XYZ_compare/6
  XY_compare/6(Zerr) -> Gain4/1
  XY_compare/5(Yerr) -> Gain5/1
  Gain5/1 -> XYZ_compare/5
  Gain3/1 -> XYZ_compare/4
  XY_compare/4(Xerr) -> Gain3/1

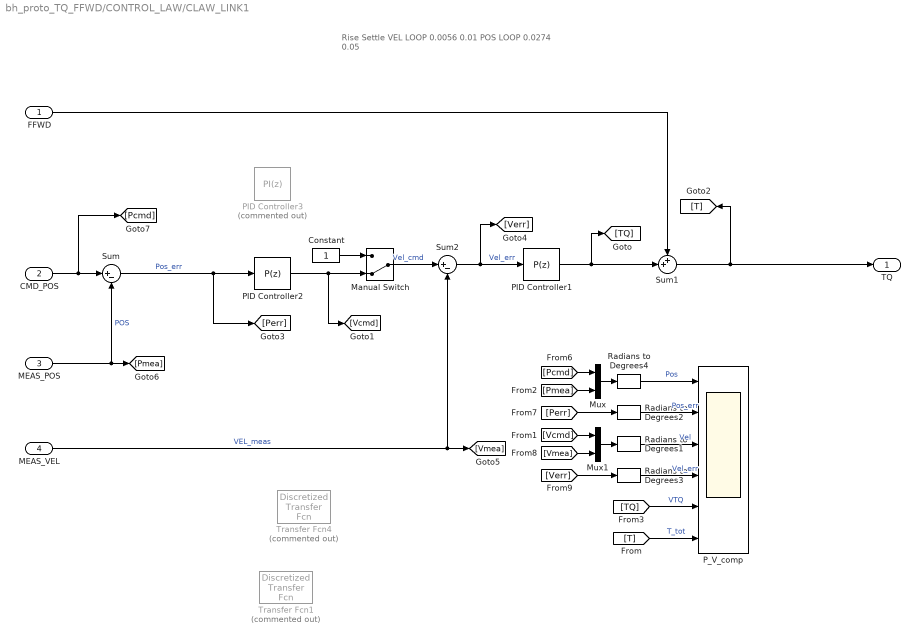
== system bh_proto_TQ_FFWD/CONTROL_LAW/CLAW_LINK1 ==
  note: Rise Settle
      | VEL LOOP 0.0056 0.01
      | POS LOOP 0.0274 0.05
  FFWD : Inport
  CMD_POS : Inport  Port=2
  MEAS_POS : Inport  Port=3
  MEAS_VEL : Inport  Port=4
  Constant : Constant
  Manual Switch : ManualSwitch  CurrentSetting=0
  Mux : Mux  Inputs=2
  Mux1 : Mux  Inputs=2
  PID Controller1 : simulink/Continuous/PID Controller  Controller=P  TimeDomain=Discrete-time  SampleTime=0.001  IntegratorMethod=Forward Euler  FilterMethod=Forward Euler  Form=Parallel  UseFilter=on  ControllerParametersSource=internal  P=91.294010645622  I=0  D=0  N=100  InitialConditionSource=internal  InitialConditionForIntegrator=0  InitialConditionForFilter=0  ExternalReset=none  LimitOutput=off  UpperSaturationLimit=inf  LowerSaturationLimit=-inf  LinearizeAsGain=on  AntiWindupMode=none  Kb=1  TrackingMode=off  Kt=1  PParamMin=[]  PParamMax=[]  IParamMin=[]  IParamMax=[]  DParamMin=[]  DParamMax=[]  NParamMin=[]  NParamMax=[]  KbParamMin=[]  KbParamMax=[]  KtParamMin=[]  KtParamMax=[]  POutMin=[]  POutMax=[]  IOutMin=[]  IOutMax=[]  DOutMin=[]  DOutMax=[]  NOutMin=[]  NOutMax=[]  KbOutMin=[]  KbOutMax=[]  KtOutMin=[]  KtOutMax=[]  IntegratorOutMin=[]  IntegratorOutMax=[]  FilterOutMin=[]  FilterOutMax=[]  SumOutMin=[]  SumOutMax=[]  SumI1OutMin=[]  SumI1OutMax=[]  SumI2OutMin=[]  SumI2OutMax=[]  SumI3OutMin=[]  SumI3OutMax=[]  SumDOutMin=[]  SumDOutMax=[]  SaturationOutMin=[]  SaturationOutMax=[]  IntegratorContinuousStateAttributes=''  IntegratorStateMustResolveToSignalObject=off  IntegratorRTWStateStorageClass=Auto  FilterContinuousStateAttributes=''  FilterStateMustResolveToSignalObject=off  FilterRTWStateStorageClass=Auto  DifferentiatorICPrevScaledInput=0  DifferentiatorOutMin=[]  DifferentiatorOutMax=[]
      settings: AttributesFormatString=DT= %<SampleTime>
  PID Controller2 : simulink/Continuous/PID Controller  Controller=P  TimeDomain=Discrete-time  SampleTime=0.001  IntegratorMethod=Forward Euler  FilterMethod=Forward Euler  Form=Parallel  UseFilter=on  ControllerParametersSource=internal  P=63.9206282980652  I=48  D=0  N=100  InitialConditionSource=internal  InitialConditionForIntegrator=0  InitialConditionForFilter=0  ExternalReset=none  LimitOutput=off  UpperSaturationLimit=inf  LowerSaturationLimit=-inf  LinearizeAsGain=on  AntiWindupMode=none  Kb=1  TrackingMode=off  Kt=1  PParamMin=[]  PParamMax=[]  IParamMin=[]  IParamMax=[]  DParamMin=[]  DParamMax=[]  NParamMin=[]  NParamMax=[]  KbParamMin=[]  KbParamMax=[]  KtParamMin=[]  KtParamMax=[]  POutMin=[]  POutMax=[]  IOutMin=[]  IOutMax=[]  DOutMin=[]  DOutMax=[]  NOutMin=[]  NOutMax=[]  KbOutMin=[]  KbOutMax=[]  KtOutMin=[]  KtOutMax=[]  IntegratorOutMin=[]  IntegratorOutMax=[]  FilterOutMin=[]  FilterOutMax=[]  SumOutMin=[]  SumOutMax=[]  SumI1OutMin=[]  SumI1OutMax=[]  SumI2OutMin=[]  SumI2OutMax=[]  SumI3OutMin=[]  SumI3OutMax=[]  SumDOutMin=[]  SumDOutMax=[]  SaturationOutMin=[]  SaturationOutMax=[]  IntegratorContinuousStateAttributes=''  IntegratorStateMustResolveToSignalObject=off  IntegratorRTWStateStorageClass=Auto  FilterContinuousStateAttributes=''  FilterStateMustResolveToSignalObject=off  FilterRTWStateStorageClass=Auto  DifferentiatorICPrevScaledInput=0  DifferentiatorOutMin=[]  DifferentiatorOutMax=[]
      settings: AttributesFormatString=DT= %<SampleTime>
  PID Controller3 : simulink/Continuous/PID Controller  Commented=on  Controller=PI  TimeDomain=Discrete-time  SampleTime=0.001  IntegratorMethod=Forward Euler  FilterMethod=Forward Euler  Form=Parallel  UseFilter=on  ControllerParametersSource=internal  P=63.9206282980652  I=48  D=0  N=100  InitialConditionSource=internal  InitialConditionForIntegrator=0  InitialConditionForFilter=0  ExternalReset=none  LimitOutput=off  UpperSaturationLimit=inf  LowerSaturationLimit=-inf  LinearizeAsGain=on  AntiWindupMode=none  Kb=1  TrackingMode=off  Kt=1  PParamMin=[]  PParamMax=[]  IParamMin=[]  IParamMax=[]  DParamMin=[]  DParamMax=[]  NParamMin=[]  NParamMax=[]  KbParamMin=[]  KbParamMax=[]  KtParamMin=[]  KtParamMax=[]  POutMin=[]  POutMax=[]  IOutMin=[]  IOutMax=[]  DOutMin=[]  DOutMax=[]  NOutMin=[]  NOutMax=[]  KbOutMin=[]  KbOutMax=[]  KtOutMin=[]  KtOutMax=[]  IntegratorOutMin=[]  IntegratorOutMax=[]  FilterOutMin=[]  FilterOutMax=[]  SumOutMin=[]  SumOutMax=[]  SumI1OutMin=[]  SumI1OutMax=[]  SumI2OutMin=[]  SumI2OutMax=[]  SumI3OutMin=[]  SumI3OutMax=[]  SumDOutMin=[]  SumDOutMax=[]  SaturationOutMin=[]  SaturationOutMax=[]  IntegratorContinuousStateAttributes=''  IntegratorStateMustResolveToSignalObject=off  IntegratorRTWStateStorageClass=Auto  FilterContinuousStateAttributes=''  FilterStateMustResolveToSignalObject=off  FilterRTWStateStorageClass=Auto  DifferentiatorICPrevScaledInput=0  DifferentiatorOutMin=[]  DifferentiatorOutMax=[]
      settings: AttributesFormatString=DT= %<SampleTime>
  P_V_comp : Scope  NumInputPorts=6
  Radians to Degrees{1..4} (4 alike) : simulink_extras/Transformations/Radians to Degrees
  Sum : Sum  Inputs=|+-
  Sum1 : Sum  Inputs=++|
  Sum2 : Sum  Inputs=|+-
  Transfer Fcn1 : discretizing/Discretized Transfer Fcn  Commented=on  Numerator=[300]  Denominator=[1 300]  AbsTol=auto  SampleTime=0.001  method=tustin  Wc=1
  Transfer Fcn4 : discretizing/Discretized Transfer Fcn  Commented=on  Numerator=[100]  Denominator=[1 100]  AbsTol=auto  SampleTime=0.001  method=tustin  Wc=1
  TQ : Outport
  wires:
  FFWD/1 -> Sum1/1
  CMD_POS/1 -> [Pcmd], Sum/1
  MEAS_VEL/1 -> [Vmea], Sum2/2  "VEL_meas"
  MEAS_POS/1 -> [Pmea], Sum/2  "POS"
  Sum2/1 -> [Verr], PID Controller1/1  "Vel_err"
  Manual Switch/1 -> Sum2/1  "Vel_cmd"
  Constant/1 -> Manual Switch/1
  Sum/1 -> PID Controller2/1, [Perr]  "Pos_err"
  PID Controller2/1 -> Manual Switch/2, [Vcmd]
  Sum1/1 -> TQ/1, [T]
  Mux/1 -> Radians to Degrees4/1
  [Pcmd] -> Mux/1
  [Pmea] -> Mux/2
  Mux1/1 -> Radians to Degrees1/1
  [Vcmd] -> Mux1/1
  [Vmea] -> Mux1/2
  [Verr] -> Radians to Degrees3/1
  [Perr] -> Radians to Degrees2/1
  Radians to Degrees3/1 -> P_V_comp/4  "Vel_err"
  Radians to Degrees2/1 -> P_V_comp/2  "Pos_err"
  Radians to Degrees1/1 -> P_V_comp/3  "Vel"
  Radians to Degrees4/1 -> P_V_comp/1  "Pos"
  [TQ] -> P_V_comp/5  "VTQ"
  [T] -> P_V_comp/6  "T_tot"
  PID Controller1/1 -> Sum1/2, [TQ]

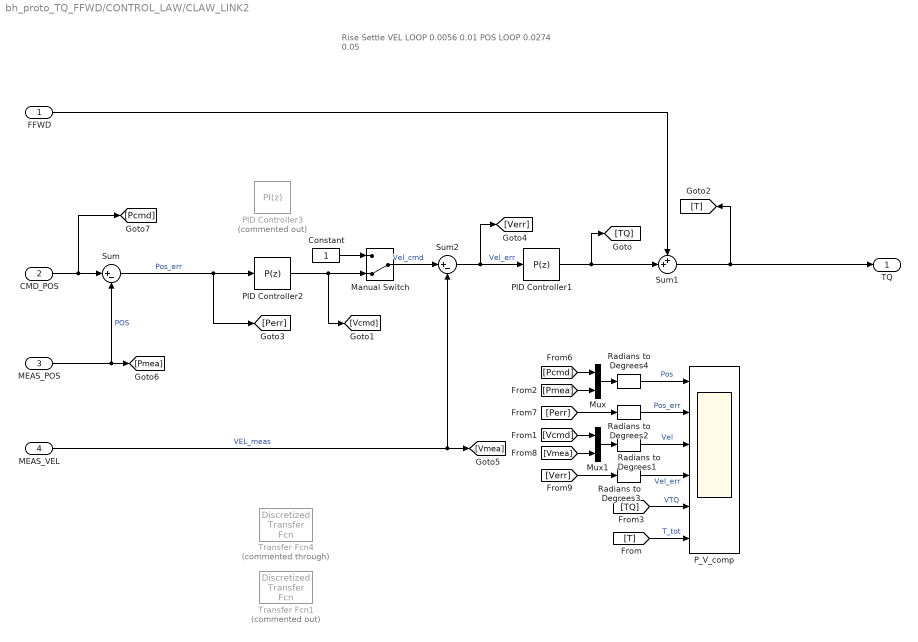
== system bh_proto_TQ_FFWD/CONTROL_LAW/CLAW_LINK2 ==
  note: Rise Settle
      | VEL LOOP 0.0056 0.01
      | POS LOOP 0.0274 0.05
  FFWD : Inport
  CMD_POS : Inport  Port=2
  MEAS_POS : Inport  Port=3
  MEAS_VEL : Inport  Port=4
  Constant : Constant
  Manual Switch : ManualSwitch  CurrentSetting=0
  Mux : Mux  Inputs=2
  Mux1 : Mux  Inputs=2
  PID Controller1 : simulink/Continuous/PID Controller  Controller=P  TimeDomain=Discrete-time  SampleTime=0.001  IntegratorMethod=Forward Euler  FilterMethod=Forward Euler  Form=Parallel  UseFilter=on  ControllerParametersSource=internal  P=12.0646813225273  I=10  D=0  N=100  InitialConditionSource=internal  InitialConditionForIntegrator=0  InitialConditionForFilter=0  ExternalReset=none  LimitOutput=off  UpperSaturationLimit=inf  LowerSaturationLimit=-inf  LinearizeAsGain=on  AntiWindupMode=none  Kb=1  TrackingMode=off  Kt=1  PParamMin=[]  PParamMax=[]  IParamMin=[]  IParamMax=[]  DParamMin=[]  DParamMax=[]  NParamMin=[]  NParamMax=[]  KbParamMin=[]  KbParamMax=[]  KtParamMin=[]  KtParamMax=[]  POutMin=[]  POutMax=[]  IOutMin=[]  IOutMax=[]  DOutMin=[]  DOutMax=[]  NOutMin=[]  NOutMax=[]  KbOutMin=[]  KbOutMax=[]  KtOutMin=[]  KtOutMax=[]  IntegratorOutMin=[]  IntegratorOutMax=[]  FilterOutMin=[]  FilterOutMax=[]  SumOutMin=[]  SumOutMax=[]  SumI1OutMin=[]  SumI1OutMax=[]  SumI2OutMin=[]  SumI2OutMax=[]  SumI3OutMin=[]  SumI3OutMax=[]  SumDOutMin=[]  SumDOutMax=[]  SaturationOutMin=[]  SaturationOutMax=[]  IntegratorContinuousStateAttributes=''  IntegratorStateMustResolveToSignalObject=off  IntegratorRTWStateStorageClass=Auto  FilterContinuousStateAttributes=''  FilterStateMustResolveToSignalObject=off  FilterRTWStateStorageClass=Auto  DifferentiatorICPrevScaledInput=0  DifferentiatorOutMin=[]  DifferentiatorOutMax=[]
      settings: AttributesFormatString=DT= %<SampleTime>
  PID Controller2 : simulink/Continuous/PID Controller  Controller=P  TimeDomain=Discrete-time  SampleTime=0.001  IntegratorMethod=Forward Euler  FilterMethod=Forward Euler  Form=Parallel  UseFilter=on  ControllerParametersSource=internal  P=1.7*64.6199485469639  I=55  D=0  N=100  InitialConditionSource=internal  InitialConditionForIntegrator=0  InitialConditionForFilter=0  ExternalReset=none  LimitOutput=off  UpperSaturationLimit=inf  LowerSaturationLimit=-inf  LinearizeAsGain=on  AntiWindupMode=none  Kb=1  TrackingMode=off  Kt=1  PParamMin=[]  PParamMax=[]  IParamMin=[]  IParamMax=[]  DParamMin=[]  DParamMax=[]  NParamMin=[]  NParamMax=[]  KbParamMin=[]  KbParamMax=[]  KtParamMin=[]  KtParamMax=[]  POutMin=[]  POutMax=[]  IOutMin=[]  IOutMax=[]  DOutMin=[]  DOutMax=[]  NOutMin=[]  NOutMax=[]  KbOutMin=[]  KbOutMax=[]  KtOutMin=[]  KtOutMax=[]  IntegratorOutMin=[]  IntegratorOutMax=[]  FilterOutMin=[]  FilterOutMax=[]  SumOutMin=[]  SumOutMax=[]  SumI1OutMin=[]  SumI1OutMax=[]  SumI2OutMin=[]  SumI2OutMax=[]  SumI3OutMin=[]  SumI3OutMax=[]  SumDOutMin=[]  SumDOutMax=[]  SaturationOutMin=[]  SaturationOutMax=[]  IntegratorContinuousStateAttributes=''  IntegratorStateMustResolveToSignalObject=off  IntegratorRTWStateStorageClass=Auto  FilterContinuousStateAttributes=''  FilterStateMustResolveToSignalObject=off  FilterRTWStateStorageClass=Auto  DifferentiatorICPrevScaledInput=0  DifferentiatorOutMin=[]  DifferentiatorOutMax=[]
      settings: AttributesFormatString=DT= %<SampleTime>
  PID Controller3 : simulink/Continuous/PID Controller  Commented=on  Controller=PI  TimeDomain=Discrete-time  SampleTime=0.001  IntegratorMethod=Forward Euler  FilterMethod=Forward Euler  Form=Parallel  UseFilter=on  ControllerParametersSource=internal  P=1.7*64.6199485469639  I=55  D=0  N=100  InitialConditionSource=internal  InitialConditionForIntegrator=0  InitialConditionForFilter=0  ExternalReset=none  LimitOutput=off  UpperSaturationLimit=inf  LowerSaturationLimit=-inf  LinearizeAsGain=on  AntiWindupMode=none  Kb=1  TrackingMode=off  Kt=1  PParamMin=[]  PParamMax=[]  IParamMin=[]  IParamMax=[]  DParamMin=[]  DParamMax=[]  NParamMin=[]  NParamMax=[]  KbParamMin=[]  KbParamMax=[]  KtParamMin=[]  KtParamMax=[]  POutMin=[]  POutMax=[]  IOutMin=[]  IOutMax=[]  DOutMin=[]  DOutMax=[]  NOutMin=[]  NOutMax=[]  KbOutMin=[]  KbOutMax=[]  KtOutMin=[]  KtOutMax=[]  IntegratorOutMin=[]  IntegratorOutMax=[]  FilterOutMin=[]  FilterOutMax=[]  SumOutMin=[]  SumOutMax=[]  SumI1OutMin=[]  SumI1OutMax=[]  SumI2OutMin=[]  SumI2OutMax=[]  SumI3OutMin=[]  SumI3OutMax=[]  SumDOutMin=[]  SumDOutMax=[]  SaturationOutMin=[]  SaturationOutMax=[]  IntegratorContinuousStateAttributes=''  IntegratorStateMustResolveToSignalObject=off  IntegratorRTWStateStorageClass=Auto  FilterContinuousStateAttributes=''  FilterStateMustResolveToSignalObject=off  FilterRTWStateStorageClass=Auto  DifferentiatorICPrevScaledInput=0  DifferentiatorOutMin=[]  DifferentiatorOutMax=[]
      settings: AttributesFormatString=DT= %<SampleTime>
  P_V_comp : Scope  NumInputPorts=6
  Radians to Degrees{1..4} (4 alike) : simulink_extras/Transformations/Radians to Degrees
  Sum : Sum  Inputs=|+-
  Sum1 : Sum  Inputs=++|
  Sum2 : Sum  Inputs=|+-
  Transfer Fcn1 : discretizing/Discretized Transfer Fcn  Commented=on  Numerator=[300]  Denominator=[1 300]  AbsTol=auto  SampleTime=0.001  method=tustin  Wc=1
  Transfer Fcn4 : discretizing/Discretized Transfer Fcn  Commented=through  Numerator=[100]  Denominator=[1 100]  AbsTol=auto  SampleTime=0.001  method=tustin  Wc=1
  TQ : Outport
  wires:
  FFWD/1 -> Sum1/1
  CMD_POS/1 -> [Pcmd], Sum/1
  MEAS_VEL/1 -> [Vmea], Sum2/2  "VEL_meas"
  MEAS_POS/1 -> [Pmea], Sum/2  "POS"
  Sum2/1 -> PID Controller1/1, [Verr]  "Vel_err"
  Manual Switch/1 -> Sum2/1  "Vel_cmd"
  Constant/1 -> Manual Switch/1
  Sum/1 -> PID Controller2/1, [Perr]  "Pos_err"
  PID Controller1/1 -> [TQ], Sum1/2
  PID Controller2/1 -> Manual Switch/2, [Vcmd]
  Sum1/1 -> TQ/1, [T]
  Mux/1 -> Radians to Degrees4/1
  [Pcmd] -> Mux/1
  [Pmea] -> Mux/2
  Mux1/1 -> Radians to Degrees1/1
  [Vcmd] -> Mux1/1
  [Vmea] -> Mux1/2
  [Verr] -> Radians to Degrees3/1
  [Perr] -> Radians to Degrees2/1
  Radians to Degrees3/1 -> P_V_comp/4  "Vel_err"
  Radians to Degrees2/1 -> P_V_comp/2  "Pos_err"
  Radians to Degrees1/1 -> P_V_comp/3  "Vel"
  Radians to Degrees4/1 -> P_V_comp/1  "Pos"
  [TQ] -> P_V_comp/5  "VTQ"
  [T] -> P_V_comp/6  "T_tot"

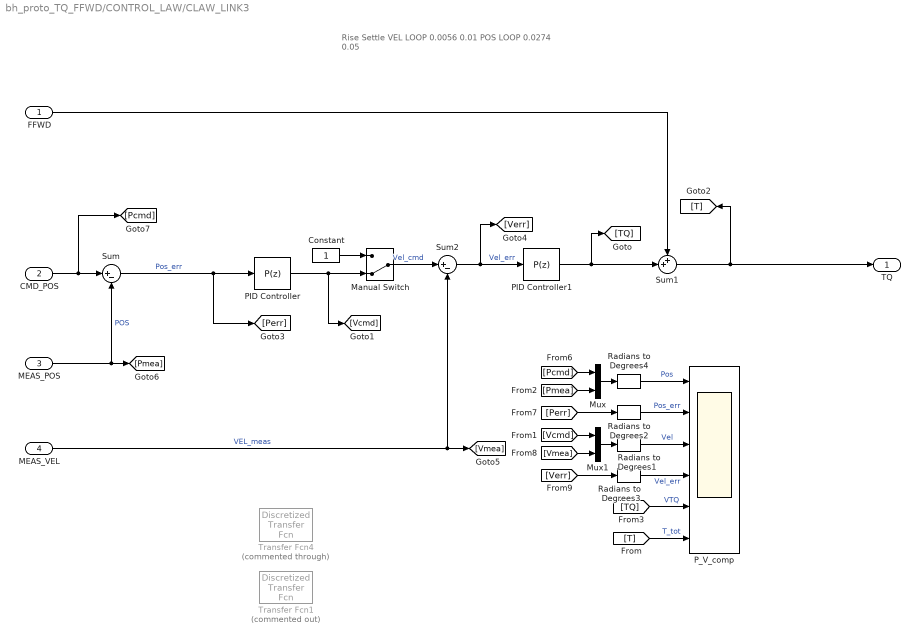
== system bh_proto_TQ_FFWD/CONTROL_LAW/CLAW_LINK3 ==
  note: Rise Settle
      | VEL LOOP 0.0056 0.01
      | POS LOOP 0.0274 0.05
  FFWD : Inport
  CMD_POS : Inport  Port=2
  MEAS_POS : Inport  Port=3
  MEAS_VEL : Inport  Port=4
  Constant : Constant
  Manual Switch : ManualSwitch  CurrentSetting=0
  Mux : Mux  Inputs=2
  Mux1 : Mux  Inputs=2
  PID Controller : simulink/Continuous/PID Controller  Controller=P  TimeDomain=Discrete-time  SampleTime=0.001  IntegratorMethod=Forward Euler  FilterMethod=Forward Euler  Form=Parallel  UseFilter=on  ControllerParametersSource=internal  P=15*4  I=20  D=0  N=100  InitialConditionSource=internal  InitialConditionForIntegrator=0  InitialConditionForFilter=0  ExternalReset=none  LimitOutput=off  UpperSaturationLimit=inf  LowerSaturationLimit=-inf  LinearizeAsGain=on  AntiWindupMode=none  Kb=1  TrackingMode=off  Kt=1  PParamMin=[]  PParamMax=[]  IParamMin=[]  IParamMax=[]  DParamMin=[]  DParamMax=[]  NParamMin=[]  NParamMax=[]  KbParamMin=[]  KbParamMax=[]  KtParamMin=[]  KtParamMax=[]  POutMin=[]  POutMax=[]  IOutMin=[]  IOutMax=[]  DOutMin=[]  DOutMax=[]  NOutMin=[]  NOutMax=[]  KbOutMin=[]  KbOutMax=[]  KtOutMin=[]  KtOutMax=[]  IntegratorOutMin=[]  IntegratorOutMax=[]  FilterOutMin=[]  FilterOutMax=[]  SumOutMin=[]  SumOutMax=[]  SumI1OutMin=[]  SumI1OutMax=[]  SumI2OutMin=[]  SumI2OutMax=[]  SumI3OutMin=[]  SumI3OutMax=[]  SumDOutMin=[]  SumDOutMax=[]  SaturationOutMin=[]  SaturationOutMax=[]  IntegratorContinuousStateAttributes=''  IntegratorStateMustResolveToSignalObject=off  IntegratorRTWStateStorageClass=Auto  FilterContinuousStateAttributes=''  FilterStateMustResolveToSignalObject=off  FilterRTWStateStorageClass=Auto  DifferentiatorICPrevScaledInput=0  DifferentiatorOutMin=[]  DifferentiatorOutMax=[]
      settings: AttributesFormatString=DT= %<SampleTime>
  PID Controller1 : simulink/Continuous/PID Controller  Controller=P  TimeDomain=Discrete-time  SampleTime=0.001  IntegratorMethod=Forward Euler  FilterMethod=Forward Euler  Form=Parallel  UseFilter=on  ControllerParametersSource=internal  P=0.422912648203834  I=10  D=0  N=100  InitialConditionSource=internal  InitialConditionForIntegrator=0  InitialConditionForFilter=0  ExternalReset=none  LimitOutput=off  UpperSaturationLimit=inf  LowerSaturationLimit=-inf  LinearizeAsGain=on  AntiWindupMode=none  Kb=1  TrackingMode=off  Kt=1  PParamMin=[]  PParamMax=[]  IParamMin=[]  IParamMax=[]  DParamMin=[]  DParamMax=[]  NParamMin=[]  NParamMax=[]  KbParamMin=[]  KbParamMax=[]  KtParamMin=[]  KtParamMax=[]  POutMin=[]  POutMax=[]  IOutMin=[]  IOutMax=[]  DOutMin=[]  DOutMax=[]  NOutMin=[]  NOutMax=[]  KbOutMin=[]  KbOutMax=[]  KtOutMin=[]  KtOutMax=[]  IntegratorOutMin=[]  IntegratorOutMax=[]  FilterOutMin=[]  FilterOutMax=[]  SumOutMin=[]  SumOutMax=[]  SumI1OutMin=[]  SumI1OutMax=[]  SumI2OutMin=[]  SumI2OutMax=[]  SumI3OutMin=[]  SumI3OutMax=[]  SumDOutMin=[]  SumDOutMax=[]  SaturationOutMin=[]  SaturationOutMax=[]  IntegratorContinuousStateAttributes=''  IntegratorStateMustResolveToSignalObject=off  IntegratorRTWStateStorageClass=Auto  FilterContinuousStateAttributes=''  FilterStateMustResolveToSignalObject=off  FilterRTWStateStorageClass=Auto  DifferentiatorICPrevScaledInput=0  DifferentiatorOutMin=[]  DifferentiatorOutMax=[]
      settings: AttributesFormatString=DT= %<SampleTime>
  P_V_comp : Scope  NumInputPorts=6
  Radians to Degrees{1..4} (4 alike) : simulink_extras/Transformations/Radians to Degrees
  Sum : Sum  Inputs=|+-
  Sum1 : Sum  Inputs=++|
  Sum2 : Sum  Inputs=|+-
  Transfer Fcn1 : discretizing/Discretized Transfer Fcn  Commented=on  Numerator=[300]  Denominator=[1 300]  AbsTol=auto  SampleTime=0.001  method=tustin  Wc=1
  Transfer Fcn4 : discretizing/Discretized Transfer Fcn  Commented=through  Numerator=[100]  Denominator=[1 100]  AbsTol=auto  SampleTime=0.001  method=tustin  Wc=1
  TQ : Outport
  wires:
  FFWD/1 -> Sum1/1
  CMD_POS/1 -> [Pcmd], Sum/1
  MEAS_VEL/1 -> [Vmea], Sum2/2  "VEL_meas"
  MEAS_POS/1 -> [Pmea], Sum/2  "POS"
  Sum2/1 -> PID Controller1/1, [Verr]  "Vel_err"
  Manual Switch/1 -> Sum2/1  "Vel_cmd"
  Constant/1 -> Manual Switch/1
  Sum/1 -> PID Controller/1, [Perr]  "Pos_err"
  PID Controller1/1 -> [TQ], Sum1/2
  PID Controller/1 -> Manual Switch/2, [Vcmd]
  Sum1/1 -> TQ/1, [T]
  Mux/1 -> Radians to Degrees4/1
  [Pcmd] -> Mux/1
  [Pmea] -> Mux/2
  Mux1/1 -> Radians to Degrees1/1
  [Vcmd] -> Mux1/1
  [Vmea] -> Mux1/2
  [Verr] -> Radians to Degrees3/1
  [Perr] -> Radians to Degrees2/1
  Radians to Degrees3/1 -> P_V_comp/4  "Vel_err"
  Radians to Degrees2/1 -> P_V_comp/2  "Pos_err"
  Radians to Degrees1/1 -> P_V_comp/3  "Vel"
  Radians to Degrees4/1 -> P_V_comp/1  "Pos"
  [TQ] -> P_V_comp/5  "VTQ"
  [T] -> P_V_comp/6  "T_tot"

== system bh_proto_TQ_FFWD/CONTROL_LAW/CLAW_LINK4 ==
  note: Rise Settle
      | VEL LOOP 0.0056 0.01
      | POS LOOP 0.0274 0.05
  FFWD : Inport
  CMD_POS : Inport  Port=2
  MEAS_POS : Inport  Port=3
  MEAS_VEL : Inport  Port=4
  Constant : Constant
  Manual Switch : ManualSwitch  CurrentSetting=0
  Mux : Mux  Inputs=2
  Mux1 : Mux  Inputs=2
  PID Controller : simulink/Continuous/PID Controller  Controller=P  TimeDomain=Discrete-time  SampleTime=0.001  IntegratorMethod=Forward Euler  FilterMethod=Forward Euler  Form=Parallel  UseFilter=on  ControllerParametersSource=internal  P=1.5*63.9206057044755  I=22  D=0  N=100  InitialConditionSource=internal  InitialConditionForIntegrator=0  InitialConditionForFilter=0  ExternalReset=none  LimitOutput=off  UpperSaturationLimit=inf  LowerSaturationLimit=-inf  LinearizeAsGain=on  AntiWindupMode=none  Kb=1  TrackingMode=off  Kt=1  PParamMin=[]  PParamMax=[]  IParamMin=[]  IParamMax=[]  DParamMin=[]  DParamMax=[]  NParamMin=[]  NParamMax=[]  KbParamMin=[]  KbParamMax=[]  KtParamMin=[]  KtParamMax=[]  POutMin=[]  POutMax=[]  IOutMin=[]  IOutMax=[]  DOutMin=[]  DOutMax=[]  NOutMin=[]  NOutMax=[]  KbOutMin=[]  KbOutMax=[]  KtOutMin=[]  KtOutMax=[]  IntegratorOutMin=[]  IntegratorOutMax=[]  FilterOutMin=[]  FilterOutMax=[]  SumOutMin=[]  SumOutMax=[]  SumI1OutMin=[]  SumI1OutMax=[]  SumI2OutMin=[]  SumI2OutMax=[]  SumI3OutMin=[]  SumI3OutMax=[]  SumDOutMin=[]  SumDOutMax=[]  SaturationOutMin=[]  SaturationOutMax=[]  IntegratorContinuousStateAttributes=''  IntegratorStateMustResolveToSignalObject=off  IntegratorRTWStateStorageClass=Auto  FilterContinuousStateAttributes=''  FilterStateMustResolveToSignalObject=off  FilterRTWStateStorageClass=Auto  DifferentiatorICPrevScaledInput=0  DifferentiatorOutMin=[]  DifferentiatorOutMax=[]
      settings: AttributesFormatString=DT= %<SampleTime>
  PID Controller1 : simulink/Continuous/PID Controller  Controller=P  TimeDomain=Discrete-time  SampleTime=0.001  IntegratorMethod=Forward Euler  FilterMethod=Forward Euler  Form=Parallel  UseFilter=on  ControllerParametersSource=internal  P=91.9060817614885  I=10  D=0  N=100  InitialConditionSource=internal  InitialConditionForIntegrator=0  InitialConditionForFilter=0  ExternalReset=none  LimitOutput=off  UpperSaturationLimit=inf  LowerSaturationLimit=-inf  LinearizeAsGain=on  AntiWindupMode=none  Kb=1  TrackingMode=off  Kt=1  PParamMin=[]  PParamMax=[]  IParamMin=[]  IParamMax=[]  DParamMin=[]  DParamMax=[]  NParamMin=[]  NParamMax=[]  KbParamMin=[]  KbParamMax=[]  KtParamMin=[]  KtParamMax=[]  POutMin=[]  POutMax=[]  IOutMin=[]  IOutMax=[]  DOutMin=[]  DOutMax=[]  NOutMin=[]  NOutMax=[]  KbOutMin=[]  KbOutMax=[]  KtOutMin=[]  KtOutMax=[]  IntegratorOutMin=[]  IntegratorOutMax=[]  FilterOutMin=[]  FilterOutMax=[]  SumOutMin=[]  SumOutMax=[]  SumI1OutMin=[]  SumI1OutMax=[]  SumI2OutMin=[]  SumI2OutMax=[]  SumI3OutMin=[]  SumI3OutMax=[]  SumDOutMin=[]  SumDOutMax=[]  SaturationOutMin=[]  SaturationOutMax=[]  IntegratorContinuousStateAttributes=''  IntegratorStateMustResolveToSignalObject=off  IntegratorRTWStateStorageClass=Auto  FilterContinuousStateAttributes=''  FilterStateMustResolveToSignalObject=off  FilterRTWStateStorageClass=Auto  DifferentiatorICPrevScaledInput=0  DifferentiatorOutMin=[]  DifferentiatorOutMax=[]
      settings: AttributesFormatString=DT= %<SampleTime>
  P_V_comp : Scope  NumInputPorts=6
  Radians to Degrees{1..4} (4 alike) : simulink_extras/Transformations/Radians to Degrees
  Sum : Sum  Inputs=|+-
  Sum1 : Sum  Inputs=++|
  Sum2 : Sum  Inputs=|+-
  Transfer Fcn1 : discretizing/Discretized Transfer Fcn  Commented=on  Numerator=[300]  Denominator=[1 300]  AbsTol=auto  SampleTime=0.001  method=tustin  Wc=1
  Transfer Fcn4 : discretizing/Discretized Transfer Fcn  Commented=through  Numerator=[100]  Denominator=[1 100]  AbsTol=auto  SampleTime=0.001  method=tustin  Wc=1
  TQ : Outport
  wires:
  FFWD/1 -> Sum1/1
  CMD_POS/1 -> [Pcmd], Sum/1
  MEAS_VEL/1 -> [Vmea], Sum2/2  "VEL_meas"
  MEAS_POS/1 -> [Pmea], Sum/2  "POS"
  Sum2/1 -> PID Controller1/1, [Verr]  "Vel_err"
  Manual Switch/1 -> Sum2/1  "Vel_cmd"
  Constant/1 -> Manual Switch/1
  Sum/1 -> PID Controller/1, [Perr]  "Pos_err"
  PID Controller1/1 -> [TQ], Sum1/2
  PID Controller/1 -> Manual Switch/2, [Vcmd]
  Sum1/1 -> TQ/1, [T]
  Mux/1 -> Radians to Degrees4/1
  [Pcmd] -> Mux/1
  [Pmea] -> Mux/2
  Mux1/1 -> Radians to Degrees1/1
  [Vcmd] -> Mux1/1
  [Vmea] -> Mux1/2
  [Verr] -> Radians to Degrees3/1
  [Perr] -> Radians to Degrees2/1
  Radians to Degrees3/1 -> P_V_comp/4  "Vel_err"
  Radians to Degrees2/1 -> P_V_comp/2  "Pos_err"
  Radians to Degrees1/1 -> P_V_comp/3  "Vel"
  Radians to Degrees4/1 -> P_V_comp/1  "Pos"
  [TQ] -> P_V_comp/5  "VTQ"
  [T] -> P_V_comp/6  "T_tot"

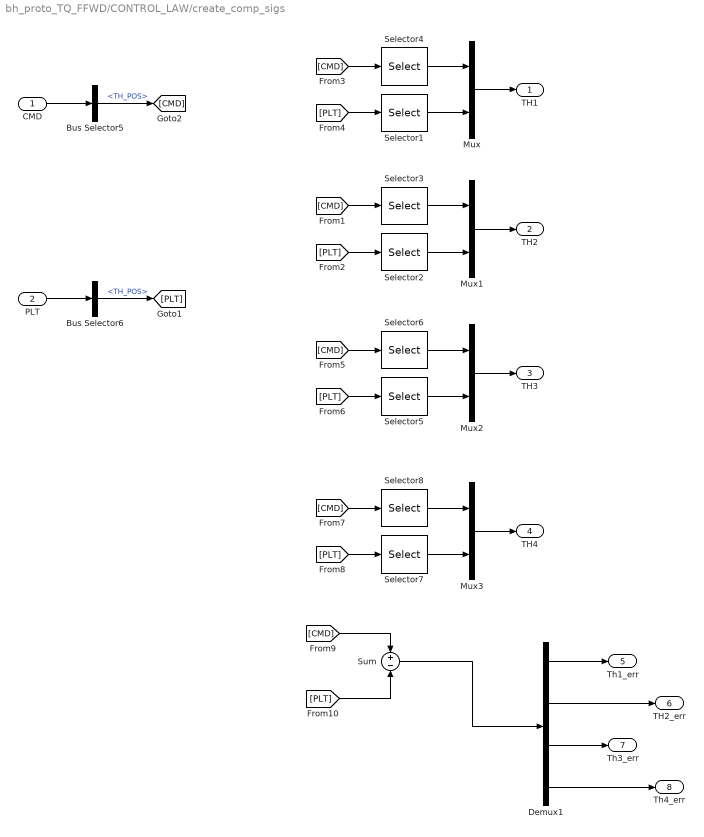
== system bh_proto_TQ_FFWD/CONTROL_LAW/create_comp_sigs ==
  CMD : Inport
  PLT : Inport  Port=2
  Bus Selector5 : BusSelector  OutputSignals=TH_POS
  Bus Selector6 : BusSelector  OutputSignals=MEAS_BUS.TH_POS
  Demux1 : Demux
  Mux{,1..3} (4 alike) : Mux  Inputs=2
  Selector1 : Selector  InputPortWidth=4  IndexOptions=Index vector (dialog)  Indices=1  OutputSizes=1
  Selector2 : Selector  InputPortWidth=4  IndexOptions=Index vector (dialog)  Indices=2  OutputSizes=1
  Selector3 : Selector  InputPortWidth=4  IndexOptions=Index vector (dialog)  Indices=2  OutputSizes=1
  Selector4 : Selector  InputPortWidth=4  IndexOptions=Index vector (dialog)  Indices=1  OutputSizes=1
  Selector5 : Selector  InputPortWidth=4  IndexOptions=Index vector (dialog)  Indices=3  OutputSizes=1
  Selector6 : Selector  InputPortWidth=4  IndexOptions=Index vector (dialog)  Indices=3  OutputSizes=1
  Selector7 : Selector  InputPortWidth=4  IndexOptions=Index vector (dialog)  Indices=4  OutputSizes=1
  Selector8 : Selector  InputPortWidth=4  IndexOptions=Index vector (dialog)  Indices=4  OutputSizes=1
  Sum : Sum  Inputs=+|-
  TH1 : Outport
  TH2 : Outport  Port=2
  TH3 : Outport  Port=3
  TH4 : Outport  Port=4
  Th1_err : Outport  Port=5
  TH2_err : Outport  Port=6
  Th3_err : Outport  Port=7
  Th4_err : Outport  Port=8
  wires:
  PLT/1 -> Bus Selector6/1
  Bus Selector6/1 -> [PLT]  "<TH_POS>"
  CMD/1 -> Bus Selector5/1
  Bus Selector5/1 -> [CMD]  "<TH_POS>"
  [CMD] -> Selector4/1
  Selector1/1 -> Mux/2
  Selector4/1 -> Mux/1
  [PLT] -> Selector1/1
  Mux/1 -> TH1/1
  [CMD] -> Selector3/1
  Selector2/1 -> Mux1/2
  Selector3/1 -> Mux1/1
  [PLT] -> Selector2/1
  Mux1/1 -> TH2/1
  [CMD] -> Selector6/1
  Selector5/1 -> Mux2/2
  Selector6/1 -> Mux2/1
  [PLT] -> Selector5/1
  Mux2/1 -> TH3/1
  [CMD] -> Selector8/1
  Selector7/1 -> Mux3/2
  Selector8/1 -> Mux3/1
  [PLT] -> Selector7/1
  Mux3/1 -> TH4/1
  [CMD] -> Sum/1
  [PLT] -> Sum/2
  Sum/1 -> Demux1/1
  Demux1/1 -> Th1_err/1
  Demux1/2 -> TH2_err/1
  Demux1/3 -> Th3_err/1
  Demux1/4 -> Th4_err/1
